simulink model "DinamicaModulo"  (R2015a)
settings: Solver=ode45  StartTime=0.0  StopTime=10.0  RelTol=1e-3
values from neighbouring files (symbols this model uses):
  J = 100000    [InitialParameters.m]
settings Model: Creator=MateusVendramini  LastModifiedBy=MateusVendramini

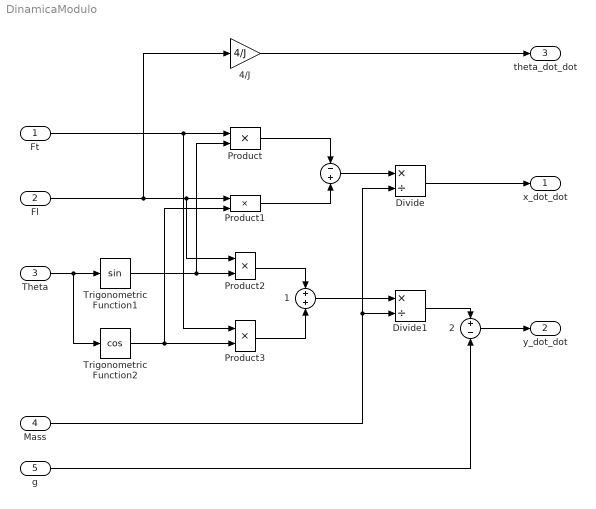
== system DinamicaModulo ==
  Ft : Inport
  Fl : Inport  Port=2
  Theta : Inport  Port=3
  "Mass " : Inport  Port=4
  "g " : Inport  Port=5
  " " : Sum  Inputs=-+
  " 1" : Sum
  " 2" : Sum  Inputs=+-
  4/J : Gain  Gain=4/J
  Divide : Product  Inputs=*/
  Divide1 : Product  Inputs=*/
  Product{,1..3} (4 alike) : Product
  Trigonometric Function1 : Trigonometry
  Trigonometric Function2 : Trigonometry  Operator=cos
  x_dot_dot : Outport
  y_dot_dot : Outport  Port=2
  theta_dot_dot : Outport  Port=3
  wires:
  Fl/1 -> 4/J/1, Product2/1, Product1/1
  Theta/1 -> Trigonometric Function2/1, Trigonometric Function1/1
  Trigonometric Function1/1 -> Product2/2, Product/2
  Trigonometric Function2/1 -> Product1/2, Product3/2
  Ft/1 -> Product/1, Product3/1
  Product1/1 -> " "/2
  Product/1 -> " "/1
  Product3/1 -> " 1"/2
  Product2/1 -> " 1"/1
  " "/1 -> Divide/1
  "Mass "/1 -> Divide1/2, Divide/2
  " 1"/1 -> Divide1/1
  Divide1/1 -> " 2"/1
  "g "/1 -> " 2"/2
  " 2"/1 -> y_dot_dot/1
  Divide/1 -> x_dot_dot/1
  4/J/1 -> theta_dot_dot/1
